simulink model "ASK"  (R2023b)
settings: Solver=VariableStepAuto  StartTime=0.0  StopTime=10.0  RelTol=1e-3
settings Model: Creator=satyamagrawal  LastModifiedBy=satyamagrawal

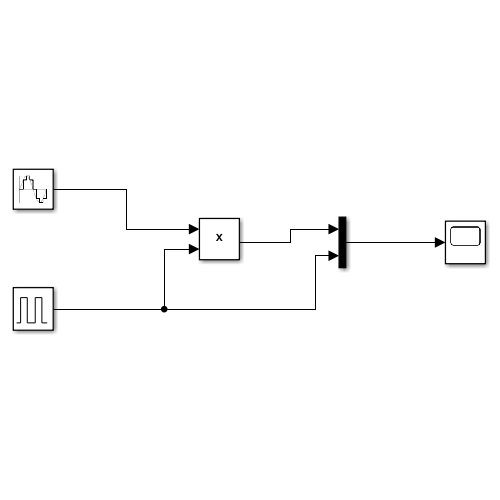
[thumbnail: Simulink's stored preview of the top-level diagram]
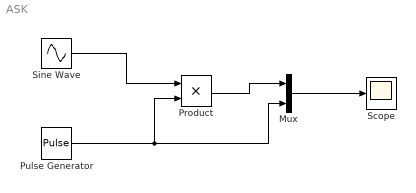
== system ASK ==
  Mux : Mux  Inputs=2
  Product : Product
  Pulse Generator : DiscretePulseGenerator  PulseType=Time based  PulseWidth=50
  Scope : Scope
  Sine Wave : Sin  Frequency=30  SampleTime=0.0001
  wires:
  Sine Wave/1 -> Product/1
  Pulse Generator/1 -> Mux/2, Product/2
  Product/1 -> Mux/1
  Mux/1 -> Scope/1
